simulink model "Real_time_2019"  (R2019b)
settings: Solver=FixedStepDiscrete  StartTime=0.0  StopTime=inf  FixedStep=0.005  RelTol=1e-3
undefined symbols (not defined in the file or in its folder): K, National_Instruments, PCI, Ts, wc
libraries: sldrtlib x2, simulink_extras x1
settings Model: SimulationMode=external  ExtModeTrigDuration=200000  Creator=magudelo  LastModifiedBy=gebruiker
settings SolverCC: InsertRTBMode=Always
settings DataIOCC: LimitDataPoints=on  SaveFormat=Array  SignalLoggingSaveFormat=ModelDataLogs  ReturnWorkspaceOutputs=off
settings OptimizationCC: ExpressionDepthLimit=2147483647
settings DebuggingCC: UnderspecifiedInitializationDetection=Classic  MergeDetectMultiDrivingBlocksExec=none  SolverPrmCheckMsg=warning  FcnCallInpInsideContextMsg=warning  StateNameClashWarn=warning  SFUnexpectedBacktrackingDiag=warning  SFNoUnconditionalDefaultTransitionDiag=warning  SFExecutionAtInitializationDiag=none  ArithmeticOperatorsInVariantConditions=warning
settings ModelReferenceCC: PropagateSignalLabelsOutOfModel=off
settings SFSimCC: SimUseLocalCustomCode=off  CustomCodeUndefinedFunction=UseInterfaceOnly
settings RTWCC: Description=Simulink Desktop Real-Time  SystemTargetFile=sldrt.tlc  TemplateMakefile=sldrt.tmf  RTWUseLocalCustomCode=off  RTWCompilerOptimization=on
settings CodeAppCC: MaxIdLength=95  StateflowObjectComments=on
settings TargetCC: TargetPreCompLibLocation=C:\Program Files\MATLAB\R2018a\toolbox\sldrt\lib\win64
settings ConfigComp: CovMetricSettings=dw  CovSaveCumulativeToWorkspaceVar=on  CovSaveSingleToWorkspaceVar=on  CovExternalEMLEnable=off

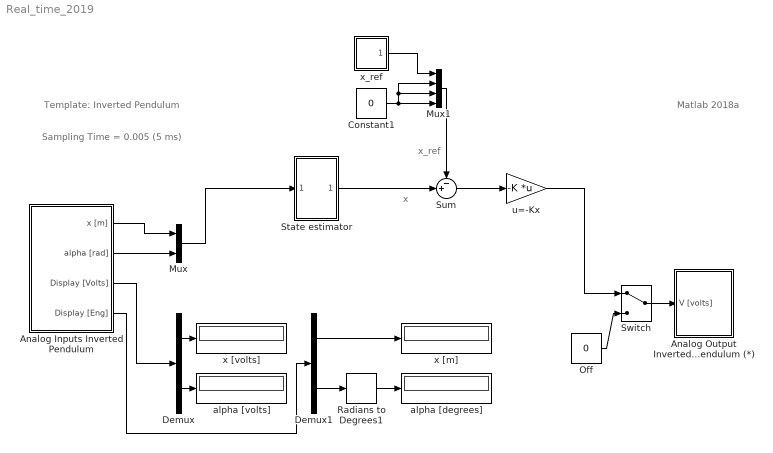
== system Real_time_2019 ==
  note: Matlab 2018a
  note: Template: Inverted Pendulum
  note: Sampling Time = 0.005 (5 ms)
  note: x_ref
  note: x
  Analog Inputs Inverted Pendulum : Subsystem  mask(Analog Inputs. Inverted Pendulum){v2m=0.1033, offset_x=0, v2r=0.2482, offset_alfa=0.17}
      mask prompts: v2m "F_x = Convertion factor from Volts to Meters:"; offset_x "Off_x = Offset for the Cart Position [Volts] :"; v2r "F_alpha = Convertion Factor from Volts to Radians :"; offset_alfa "Off_alpha = Offset for the angle of the rob [Volts] :"
      mask help:
      | Remember:
      |    Cart Position (x)           => channel ACH0
      |    Angle of the rod (alpha) => channel ACH1
      |
      |   Cart Position [m] = F_x * ( Cart Position [v] + off_x )
      |   Angle of the rod [rad] = F_alpha * ( Angle of the rod [v] + off_alpha )
  Analog Output Inverted Pendulum (*) : Subsystem  mask(Analog Output - Inverted Pendulum){}
      mask help:
      | Remember
      |    AO 0 => Power Amplifier + Motor
  Constant1 : Constant  Value=0
  Demux : Demux  Outputs=2
  Demux1 : Demux  Outputs=2
  Mux : Mux  Inputs=2
  Mux1 : Mux
  Off : Constant  Value=0
  Radians to Degrees1 : simulink_extras/Transformations/Radians to Degrees
  State estimator : Subsystem
  Sum : Sum  Inputs=-+|
  "Switch  " : ManualSwitch
  alpha [degrees] : Display
  alpha [volts] : Display
  u=-Kx : Gain  Gain=-K  Multiplication=Matrix(K*u)
  x [m] : Display
  x [volts] : Display
  x_ref : Subsystem
  wires:
  Off/1 -> "Switch  "/2
  "Switch  "/1 -> Analog Output Inverted Pendulum (*)/1(V [volts])
  Demux/1 -> x [volts]/1
  Demux1/1 -> x [m]/1
  Demux1/2 -> Radians to Degrees1/1
  Radians to Degrees1/1 -> alpha [degrees]/1
  Analog Inputs Inverted Pendulum/4(Display [Eng]) -> Demux1/1
  Demux/2 -> alpha [volts]/1
  Analog Inputs Inverted Pendulum/3(Display [Volts]) -> Demux/1
  Analog Inputs Inverted Pendulum/2(alpha [rad]) -> Mux/2
  Analog Inputs Inverted Pendulum/1(x [m]) -> Mux/1
  x_ref/1(Out1) -> Mux1/1
  u=-Kx/1 -> "Switch  "/1
  Sum/1 -> u=-Kx/1
  Mux1/1 -> Sum/1
  Constant1/1 -> Mux1/2, Mux1/3, Mux1/4
  State estimator/1(Out1) -> Sum/2
  Mux/1 -> State estimator/1(In1)

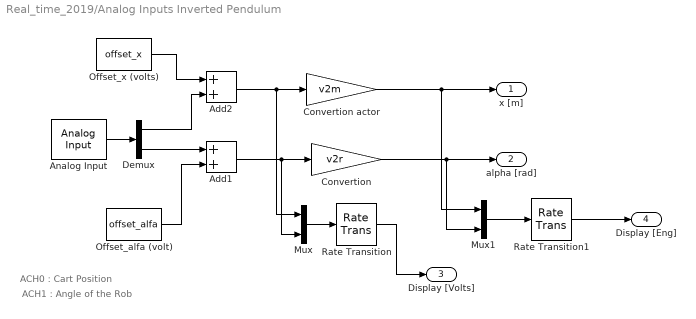
== system Real_time_2019/Analog Inputs Inverted Pendulum ==
  note: ACH0 : Cart Position
  note: ACH1 : Angle of the Rob
  Add1 : Sum
  Add2 : Sum
  Analog Input : sldrtlib/Analog Input  SampleTime=0.005  MaxMissedTicks=10  ShowMissedTicks=off  YieldWhenWaiting=off  DrvName=National_Instruments/PCI-6014  DrvAddress=4294967295  DrvOptions=[1 0 0 0 0 0]  Channels=[1 2]  RangeMode=1  VoltRange=1  DataType=1
      settings: AttributesFormatString=National Instruments\nPCI-6014 [auto]
  "Convertion " : Gain  Gain=v2r
  Convertion actor : Gain  Gain=v2m
  Demux : Demux  Outputs=2
  Mux : Mux  Inputs=2
  Mux1 : Mux  Inputs=2
  Offset_alfa (volt) : Constant  Value=offset_alfa
  Offset_x (volts) : Constant  Value=offset_x
  Rate Transition : RateTransition  OutPortSampleTime=0.25
  Rate Transition1 : RateTransition  OutPortSampleTime=0.25
  x [m] : Outport  VectorParamsAs1DForOutWhenUnconnected=off
  alpha [rad] : Outport  Port=2  VectorParamsAs1DForOutWhenUnconnected=off
  Display [Volts] : Outport  Port=3  VectorParamsAs1DForOutWhenUnconnected=off
  Display [Eng] : Outport  Port=4  VectorParamsAs1DForOutWhenUnconnected=off
  wires:
  Analog Input/1 -> Demux/1
  Demux/1 -> Add2/2
  Add2/1 -> Convertion actor/1, Mux/1
  Offset_x (volts)/1 -> Add2/1
  Convertion actor/1 -> x [m]/1, Mux1/1
  Demux/2 -> Add1/1
  Offset_alfa (volt)/1 -> Add1/2
  Add1/1 -> "Convertion "/1, Mux/2
  "Convertion "/1 -> alpha [rad]/1, Mux1/2
  Mux/1 -> Rate Transition/1
  Rate Transition/1 -> Display [Volts]/1
  Mux1/1 -> Rate Transition1/1
  Rate Transition1/1 -> Display [Eng]/1

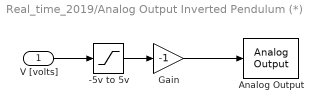
== system Real_time_2019/Analog Output Inverted Pendulum (*) ==
  V [volts] : Inport
  -5v to 5v : Saturate  UpperLimit=5  LowerLimit=-5
  Analog Output : sldrtlib/Analog Output  SampleTime=0.005  MaxMissedTicks=10  ShowMissedTicks=off  YieldWhenWaiting=off  DrvName=National_Instruments/PCI-6014  DrvAddress=4294967295  DrvOptions=[1 0 0 0 0 0]  Channels=1  RangeMode=1  VoltRange=1  InitialValue=0  FinalValue=0
      settings: AttributesFormatString=National Instruments\nPCI-6014 [auto]
  Gain : Gain  Gain=-1
  wires:
  -5v to 5v/1 -> Gain/1
  V [volts]/1 -> -5v to 5v/1
  Gain/1 -> Analog Output/1

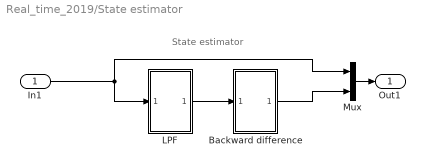
== system Real_time_2019/State estimator ==
  note: State estimator
  In1 : Inport
  Backward difference : Subsystem
  LPF : Subsystem
  Mux : Mux  Inputs=2
  Out1 : Outport
  wires:
  LPF/1(Out1) -> Backward difference/1(In1)
  Backward difference/1(Out1) -> Mux/2
  Mux/1 -> Out1/1
  In1/1 -> Mux/1, LPF/1(In1)

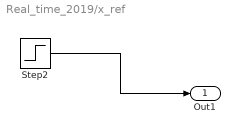
== system Real_time_2019/x_ref ==
  Step2 : Step  SampleTime=0
  Out1 : Outport
  wires:
  Step2/1 -> Out1/1

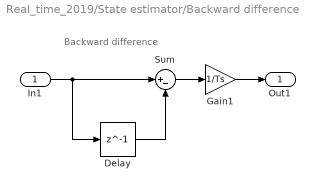
== system Real_time_2019/State estimator/Backward difference ==
  note: Backward difference
  In1 : Inport
  Delay : Delay  DelayLength=1  InitialCondition=0
  Gain1 : Gain  Gain=1/Ts
  Sum : Sum  Inputs=|+-
  Out1 : Outport
  wires:
  Delay/1 -> Sum/2
  Gain1/1 -> Out1/1
  In1/1 -> Delay/1, Sum/1
  Sum/1 -> Gain1/1

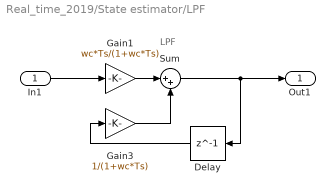
== system Real_time_2019/State estimator/LPF ==
  note: LPF
  In1 : Inport
  Delay : Delay  DelayLength=1
  Gain1 : Gain  Gain=wc*Ts/(1+wc*Ts)
  Gain3 : Gain  Gain=1/(1+wc*Ts)
  Sum : Sum  Inputs=|++
  Out1 : Outport
  wires:
  Gain3/1 -> Sum/2
  Sum/1 -> Out1/1, Delay/1
  Delay/1 -> Gain3/1
  In1/1 -> Gain1/1
  Gain1/1 -> Sum/1
